simulink model "UnicycleAccModel_wPatch_2024b"  (R2024b)
settings: Solver=VariableStepAuto  StartTime=0.0  StopTime=10.0  RelTol=1e-3
PostLoadFcn:
  | run("parameters.m")
InitFcn:
  | run("parameters.m")
StartFcn:
  | run("parameters.m")
values from neighbouring files (symbols this model uses):
  a = 1000    [combined.mat]    (also in parameters_combined.m)
  delta = 1    [combined.mat]    (also in parameters_combined.m)
  k1_reg = 1.2    [combined.mat]    (also in parameters_combined.m)
  k2_reg = 0.7    [combined.mat]    (also in parameters_combined.m)
  k3_reg = 0.1    [combined.mat]    (also in parameters_combined.m)
  ksi = 0.5    [combined.mat]    (also in parameters_combined.m)
  wc = 0.314159265359    [combined.mat]    (also in parameters_combined.m)
libraries: SignalEditorBlockLib x2
settings Model: Creator=federico  LastModifiedBy=aboulenien

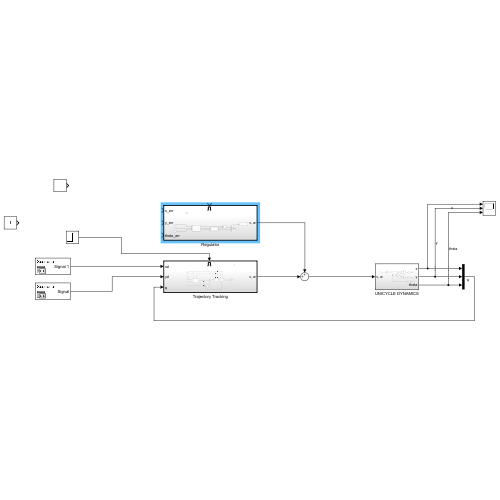
[thumbnail: Simulink's stored preview of the top-level diagram]
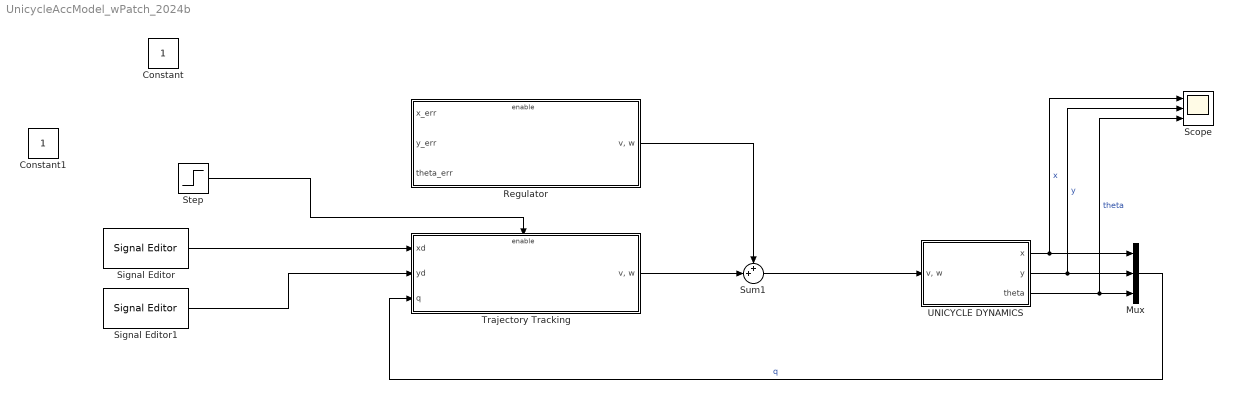
== system UnicycleAccModel_wPatch_2024b ==
  Constant : Constant
  Constant1 : Constant
  Mux : Mux  Inputs=3
  Regulator : Subsystem  TreatAsAtomicUnit=on
  Scope : Scope  NumInputPorts=3
  Signal Editor : SignalEditorBlockLib/Signal Editor  FileName=test_1.mat  ActiveScenario=Scenario  ActiveSignal=Signal 1  IsBus=off  OutputBusObjectStr=Bus: BusObject  SampleTime=0  Interpolate=off  ZeroCross=off  OutputAfterFinalValue=Setting to zero  Unit=inherit  PreserveSignalName=on  ApplySigPropsToAllScenarios=on  ApplySigPropsToAllSignals=off
  Signal Editor1 : SignalEditorBlockLib/Signal Editor  FileName=test_1_y.mat  ActiveScenario=Scenario  ActiveSignal=Signal  IsBus=off  OutputBusObjectStr=Bus: BusObject  SampleTime=0  Interpolate=off  ZeroCross=off  OutputAfterFinalValue=Setting to zero  Unit=inherit  PreserveSignalName=on  ApplySigPropsToAllScenarios=on  ApplySigPropsToAllSignals=off
  Step : Step  Time=0  SampleTime=0
  Sum1 : Sum  Inputs=++|
  Trajectory Tracking : Subsystem
  UNICYCLE DYNAMICS : Subsystem
  wires:
  UNICYCLE DYNAMICS/1(x) -> Scope/1, Mux/1  "x"
  UNICYCLE DYNAMICS/2(y) -> Scope/2, Mux/2  "y"
  UNICYCLE DYNAMICS/3(theta) -> Scope/3, Mux/3  "theta"
  Mux/1 -> Trajectory Tracking/3(q)  "q"
  Trajectory Tracking/1("v, w") -> Sum1/2
  Sum1/1 -> UNICYCLE DYNAMICS/1("v, w")
  Regulator/1("v, w") -> Sum1/1
  Signal Editor/1 -> Trajectory Tracking/1(xd)
  Signal Editor1/1 -> Trajectory Tracking/2(yd)
  Step/1 -> Trajectory Tracking/Enable

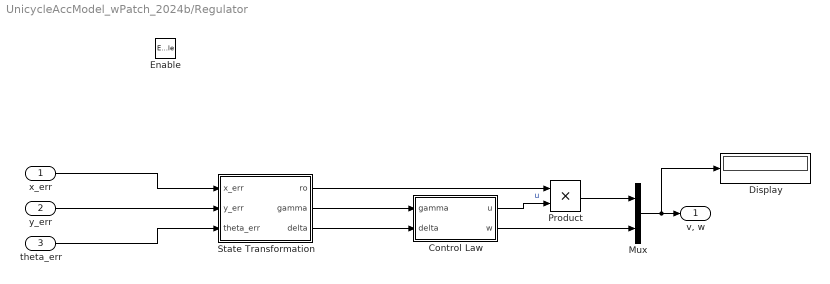
== system UnicycleAccModel_wPatch_2024b/Regulator ==
  x_err : Inport
  y_err : Inport  Port=2
  theta_err : Inport  Port=3
  Enable : EnablePort  StatesWhenEnabling=reset
  Control Law : Subsystem
  Display : Display
  Mux : Mux  Inputs=2
  Product : Product
  State Transformation : Subsystem
  "v, w" : Outport  OutputWhenDisabled=reset  InitialOutput=[0]
  wires:
  x_err/1 -> State Transformation/1(x_err)
  y_err/1 -> State Transformation/2(y_err)
  theta_err/1 -> State Transformation/3(theta_err)
  State Transformation/2(gamma) -> Control Law/1(gamma)
  State Transformation/3(delta) -> Control Law/2(delta)
  Control Law/1(u) -> Product/2  "u"
  State Transformation/1(ro) -> Product/1
  Product/1 -> Mux/1
  Control Law/2(w) -> Mux/2
  Mux/1 -> Display/1, "v, w"/1

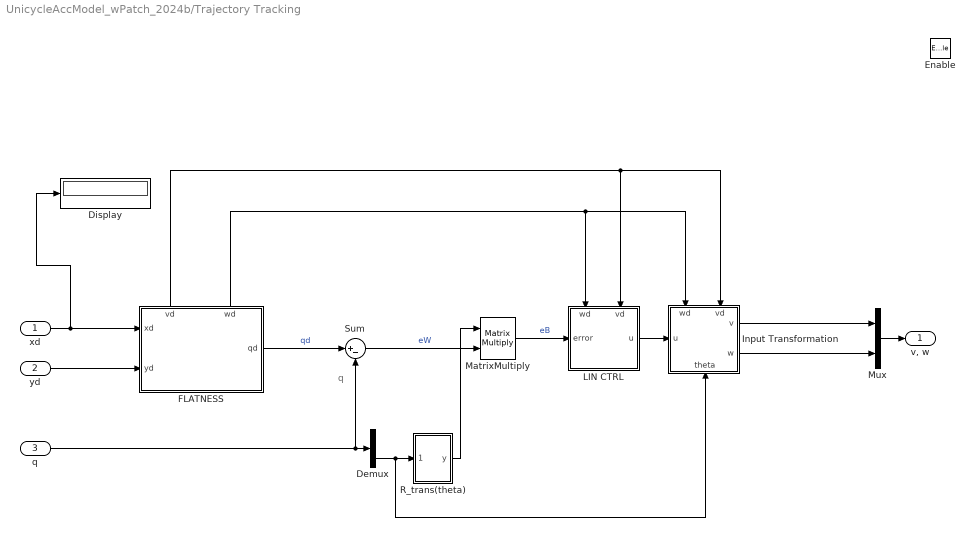
== system UnicycleAccModel_wPatch_2024b/Trajectory Tracking ==
  note: q
  xd : Inport
  yd : Inport  Port=2
  q : Inport  Port=3
  Enable : EnablePort  StatesWhenEnabling=reset
  Demux : Demux  Outputs=3
  Display : Display
  FLATNESS : Subsystem
      settings: PortSchema="{\"entries\":[{\"content\":{\"sides\":[{\"content\":{\"connectorIds\":[\"In1\",\"In2\"]},\"type\":\"ConnectorPlacement.EquallySpacedRectSide\",\"uuid\":\"cea3e210-9f99-4e4d-8873-7e28fd5d94f8\"},{\"content\":{\"connectorIds\":[\"Out1\"],\"side\":\"RIGHT\"},\"type\":\"ConnectorPlacement.EquallySpacedRectSide\",\"uuid\":\"8647a18a-6d48-4042-ba10-3487ed160766\"},{\"content\":{\"connectorIds\":[\"Out2\",\"Out3\"],\"side\":\"TOP\"},\"type\":\"ConnectorPlacement.EquallySpacedRectSide\",\"uuid\":\"5d316579-2966-4167-b423-a888f6131fb8\"}]},\"type\":\"ConnectorPlacement.EquallySpacedConnector\",\"uuid\":\"245bddfc-2899-40ea-8a56-579c88903fee\"}],\"packageUris\":[\"http://schema.mathworks.com/mf0/Connector/R2020b\"],\"version\":\"1.0\"}"
  Input Transformation : Subsystem
      settings: PortSchema="{\"entries\":[{\"content\":{\"sides\":[{\"content\":{\"connectorIds\":[\"In1\"]},\"type\":\"ConnectorPlacement.EquallySpacedRectSide\",\"uuid\":\"62ce4f7f-2237-41e7-81ad-cc04387003fd\"},{\"content\":{\"connectorIds\":[\"Out1\",\"Out2\"],\"side\":\"RIGHT\"},\"type\":\"ConnectorPlacement.EquallySpacedRectSide\",\"uuid\":\"6ba9cac5-01e4-4ff8-8743-78e2d9981801\"},{\"content\":{\"connectorIds\":[\"In2\",\"In3\"],\"side\":\"TOP\"},\"type\":\"ConnectorPlacement.EquallySpacedRectSide\",\"uuid\":\"b18d3054-a075-4e7c-bb98-889ca19f4186\"},{\"content\":{\"connectorIds\":[\"In4\"],\"side\":\"BOTTOM\"},\"type\":\"ConnectorPlacement.EquallySpacedRectSide\",\"uuid\":\"bfd13203-cad3-4607-bd21-5da97b33eddc\"}]},\"type\":\"ConnectorPlacement.EquallySpacedConnector\",\"uuid\":\"5c2e42c9-72a9-4057-8329-3756e6e7609e\"}],\"packageUris\":[\"http://schema.mathworks.com/mf0/Connector/R2020b\"],\"version\":\"1.0\"}"
  LIN CTRL : Subsystem
      settings: PortSchema="{\"entries\":[{\"content\":{\"sides\":[{\"content\":{\"connectorIds\":[\"In1\"]},\"type\":\"ConnectorPlacement.EquallySpacedRectSide\",\"uuid\":\"07dbe3dc-a27c-4138-9c4e-e0d75778e148\"},{\"content\":{\"connectorIds\":[\"Out1\"],\"side\":\"RIGHT\"},\"type\":\"ConnectorPlacement.EquallySpacedRectSide\",\"uuid\":\"18cdcdab-8a0b-458a-bb96-9cb1aca38d27\"},{\"content\":{\"connectorIds\":[\"In2\",\"In3\"],\"side\":\"TOP\"},\"type\":\"ConnectorPlacement.EquallySpacedRectSide\",\"uuid\":\"c2fd7b24-aaa4-4c4a-8e5b-04ff8b53c255\"}]},\"type\":\"ConnectorPlacement.EquallySpacedConnector\",\"uuid\":\"92e13242-08a3-4561-886e-cae250b2f145\"}],\"packageUris\":[\"http://schema.mathworks.com/mf0/Connector/R2020b\"],\"version\":\"1.0\"}"
  MatrixMultiply : Product  Multiplication=Matrix(*)
  Mux : Mux  Inputs=2
  R_trans(theta) : MATLAB Function  TreatAsAtomicUnit=on
  Sum : Sum  Inputs=|+-
  "v, w" : Outport  OutputWhenDisabled=reset  InitialOutput=[0]
  wires:
  Demux/3 -> Input Transformation/4(theta), R_trans(theta)/1(theta)
  FLATNESS/2(vd) -> Input Transformation/3(vd), LIN CTRL/3(vd)
  LIN CTRL/1(u) -> Input Transformation/1(u)
  FLATNESS/3(wd) -> Input Transformation/2(wd), LIN CTRL/2(wd)
  Sum/1 -> MatrixMultiply/2  "eW"
  FLATNESS/1(qd) -> Sum/1  "qd"
  R_trans(theta)/1(y) -> MatrixMultiply/1
  MatrixMultiply/1 -> LIN CTRL/1(error)  "eB"
  Input Transformation/2(w) -> Mux/2
  q/1 -> Demux/1, Sum/2
  yd/1 -> FLATNESS/2(yd)
  xd/1 -> Display/1, FLATNESS/1(xd)
  Mux/1 -> "v, w"/1
  Input Transformation/1(v) -> Mux/1

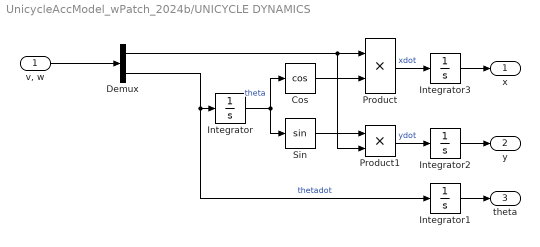
== system UnicycleAccModel_wPatch_2024b/UNICYCLE DYNAMICS ==
  "v, w" : Inport
  Cos : Trigonometry  Operator=cos
  Demux : Demux  Outputs=2
  Integrator : Integrator
  Integrator1 : Integrator
  Integrator2 : Integrator  InitialCondition=50
  Integrator3 : Integrator  InitialCondition=100
  Product : Product
  Product1 : Product
  Sin : Trigonometry
  x : Outport
  y : Outport  Port=2
  theta : Outport  Port=3
  wires:
  Demux/2 -> Integrator1/1, Integrator/1  "thetadot"
  Product/1 -> Integrator3/1  "xdot"
  Sin/1 -> Product1/1
  Product1/1 -> Integrator2/1  "ydot"
  Integrator/1 -> Sin/1, Cos/1  "theta"
  Cos/1 -> Product/2
  Integrator3/1 -> x/1
  Integrator2/1 -> y/1
  Integrator1/1 -> theta/1
  "v, w"/1 -> Demux/1
  Demux/1 -> Product1/2, Product/1

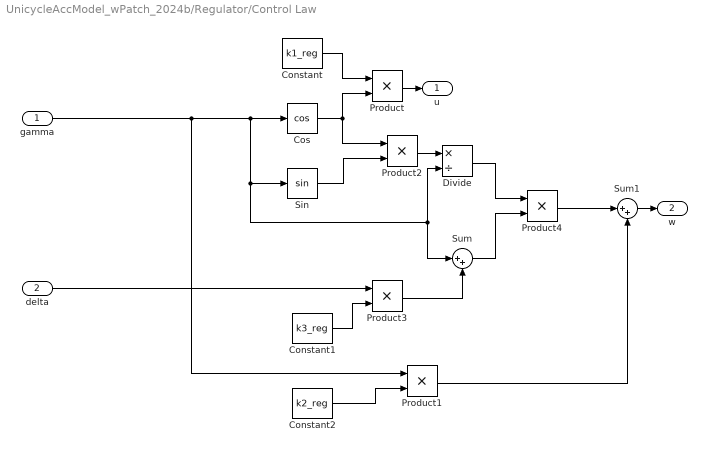
== system UnicycleAccModel_wPatch_2024b/Regulator/Control Law ==
  gamma : Inport
  delta : Inport  Port=2
  Constant : Constant  Value=k1_reg
  Constant1 : Constant  Value=k3_reg
  Constant2 : Constant  Value=k2_reg
  Cos : Trigonometry  Operator=cos
  Divide : Product  Inputs=*/
  Product{,1..4} (5 alike) : Product
  Sin : Trigonometry
  Sum : Sum  Inputs=|++
  Sum1 : Sum  Inputs=|++
  u : Outport
  w : Outport  Port=2
  wires:
  Divide/1 -> Product4/1
  Sum1/1 -> w/1
  gamma/1 -> Product1/1, Sum/1, Divide/2, Sin/1, Cos/1
  Cos/1 -> Product2/1, Product/2
  Product2/1 -> Divide/1
  Product1/1 -> Sum1/2
  Constant/1 -> Product/1
  Constant1/1 -> Product3/2
  Product3/1 -> Sum/2
  delta/1 -> Product3/1
  Sum/1 -> Product4/2
  Constant2/1 -> Product1/2
  Sin/1 -> Product2/2
  Product/1 -> u/1
  Product4/1 -> Sum1/1

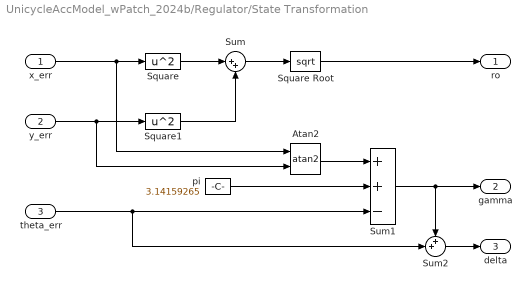
== system UnicycleAccModel_wPatch_2024b/Regulator/State Transformation ==
  x_err : Inport
  y_err : Inport  Port=2
  theta_err : Inport  Port=3
  Atan2 : Trigonometry  Operator=atan2
  Square : Math  Operator=square
  Square Root : Sqrt
  Square1 : Math  Operator=square
  Sum : Sum  Inputs=|++
  Sum1 : Sum  Inputs=++-
  Sum2 : Sum  Inputs=++|
  pi : Constant  Value=3.14159265
  ro : Outport
  gamma : Outport  Port=2
  delta : Outport  Port=3
  wires:
  Sum1/1 -> gamma/1, Sum2/1
  Sum/1 -> Square Root/1
  y_err/1 -> Atan2/2, Square1/1
  pi/1 -> Sum1/2
  Atan2/1 -> Sum1/1
  x_err/1 -> Atan2/1, Square/1
  Square Root/1 -> ro/1
  Square1/1 -> Sum/2
  Square/1 -> Sum/1
  theta_err/1 -> Sum2/2, Sum1/3
  Sum2/1 -> delta/1

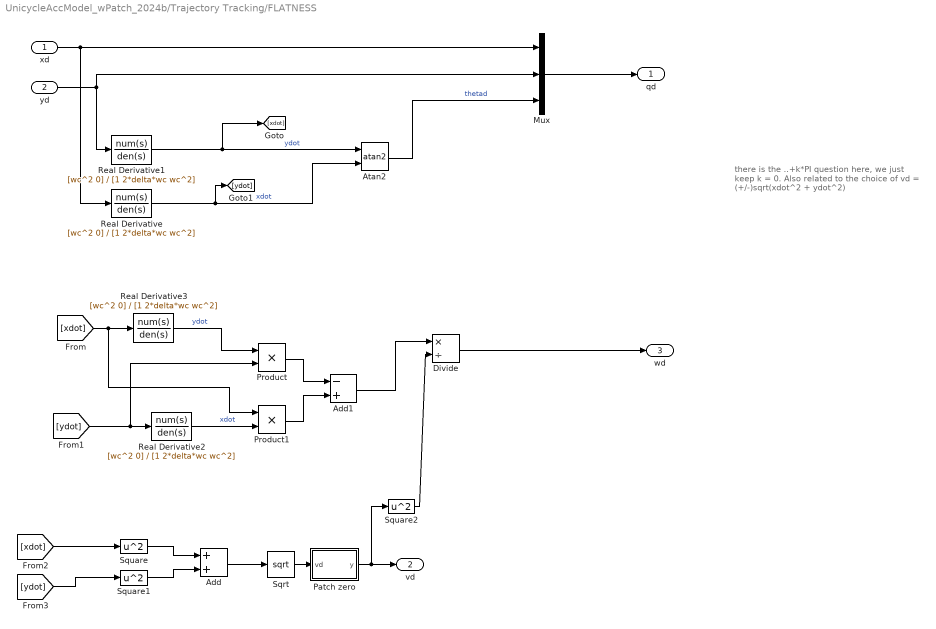
== system UnicycleAccModel_wPatch_2024b/Trajectory Tracking/FLATNESS ==
  note: there is the ..+k*PI question here,
      | we just keep k = 0.
      | Also related to the choice of
      | vd = (+/-)sqrt(xdot^2 + ydot^2)
  xd : Inport
  yd : Inport  Port=2
  Add : Sum
  Add1 : Sum  Inputs=-+
  Atan2 : Trigonometry  Operator=atan2
  Divide : Product  Inputs=*/
  Mux : Mux  Inputs=3
  Patch zero : MATLAB Function  TreatAsAtomicUnit=on
  Product : Product
  Product1 : Product
  Real Derivative{,1..3} (4 alike) : TransferFcn  Numerator=[wc^2 0]  Denominator=[1 2*delta*wc wc^2]
  Sqrt : Sqrt
  Square : Math  Operator=square
  Square1 : Math  Operator=square
  Square2 : Math  Operator=square
  qd : Outport
  vd : Outport  Port=2
  wd : Outport  Port=3
  wires:
  xd/1 -> Mux/1, Real Derivative/1
  yd/1 -> Mux/2, Real Derivative1/1
  Mux/1 -> qd/1
  Real Derivative1/1 -> [xdot], Atan2/1  "ydot"
  Real Derivative/1 -> [ydot], Atan2/2  "xdot"
  Atan2/1 -> Mux/3  "thetad"
  Add/1 -> Sqrt/1
  Square/1 -> Add/1
  Square1/1 -> Add/2
  [xdot] -> Product1/1, Real Derivative3/1
  [ydot] -> Product/2, Real Derivative2/1
  Real Derivative3/1 -> Product/1  "ydot"
  Real Derivative2/1 -> Product1/2  "xdot"
  Product/1 -> Add1/1
  Product1/1 -> Add1/2
  [xdot] -> Square/1
  [ydot] -> Square1/1
  Add1/1 -> Divide/1
  Divide/1 -> wd/1
  Sqrt/1 -> Patch zero/1(vd)
  Patch zero/1(y) -> Square2/1, vd/1
  Square2/1 -> Divide/2

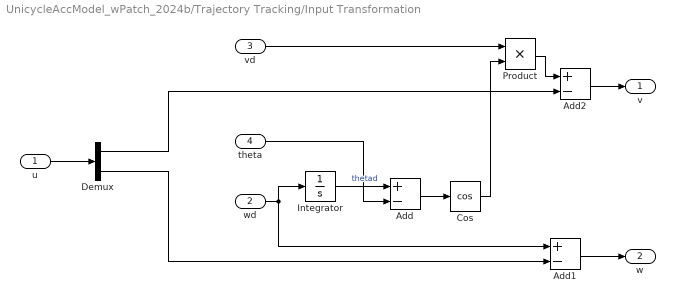
== system UnicycleAccModel_wPatch_2024b/Trajectory Tracking/Input Transformation ==
  u : Inport
  wd : Inport  Port=2
  vd : Inport  Port=3
  theta : Inport  Port=4
  Add : Sum  Inputs=+-
  Add1 : Sum  Inputs=+-
  Add2 : Sum  Inputs=+-
  Cos : Trigonometry  Operator=cos
  Demux : Demux  Outputs=2
  Integrator : Integrator
  Product : Product
  v : Outport
  w : Outport  Port=2
  wires:
  wd/1 -> Add1/1, Integrator/1
  Integrator/1 -> Add/1  "thetad"
  theta/1 -> Add/2
  Add/1 -> Cos/1
  Add1/1 -> w/1
  Demux/2 -> Add1/2
  vd/1 -> Product/1
  Cos/1 -> Product/2
  Demux/1 -> Add2/2
  Product/1 -> Add2/1
  Add2/1 -> v/1
  u/1 -> Demux/1

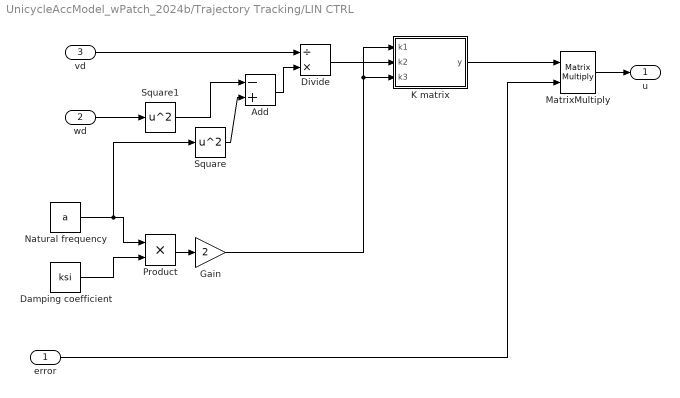
== system UnicycleAccModel_wPatch_2024b/Trajectory Tracking/LIN CTRL ==
  error : Inport
  wd : Inport  Port=2
  vd : Inport  Port=3
  Add : Sum  Inputs=-+
  Damping coefficient : Constant  Value=ksi
  Divide : Product  Inputs=/*
  Gain : Gain  Gain=2
  K matrix : MATLAB Function  TreatAsAtomicUnit=on
  MatrixMultiply : Product  Multiplication=Matrix(*)
  Natural frequency : Constant  Value=a
  Product : Product
  Square : Math  Operator=square
  Square1 : Math  Operator=square
  u : Outport
  wires:
  K matrix/1(y) -> MatrixMultiply/1
  Natural frequency/1 -> Square/1, Product/1
  Damping coefficient/1 -> Product/2
  Product/1 -> Gain/1
  wd/1 -> Square1/1
  Square1/1 -> Add/1
  Square/1 -> Add/2
  Add/1 -> Divide/2
  Divide/1 -> K matrix/2(k2)
  Gain/1 -> K matrix/1(k1), K matrix/3(k3)
  error/1 -> MatrixMultiply/2
  MatrixMultiply/1 -> u/1
  vd/1 -> Divide/1

== matlab function UnicycleAccModel_wPatch_2024b/Trajectory Tracking/LIN CTRL/K matrix ==
  data: y output; k1 input; k2 input; k3 input
function y = fcn(k1, k2, k3)

K = [-k1 0 0;...
    0 -k2 -k3];

y = K;

== matlab function UnicycleAccModel_wPatch_2024b/Trajectory Tracking/R_trans(theta) ==
  data: theta input; y output
function y = fcn(theta)
R = [cos(theta) sin(theta) 0;...
    -sin(theta) cos(theta) 0;...
    0 0 1];
y = R;

== matlab function UnicycleAccModel_wPatch_2024b/Trajectory Tracking/FLATNESS/Patch zero ==
  data: vd input; y output
function y = fcn(vd)

vd = vd;


if abs(vd) < 1e-4
    if vd >= 0
        vd = 1e-4;
    else
        vd = -1e-4;
    end
end

y = vd;
